simulink model "esquemasi"  (R2020a)
settings: Solver=VariableStepAuto  StartTime=0.0  StopTime=inf  RelTol=1e-3
libraries: simulink x1
settings Model: Creator=TATTO PC  LastModifiedBy=TATTO PC

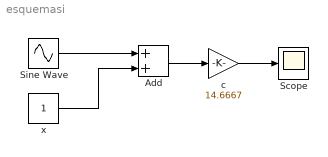
== system esquemasi ==
  Add : Sum
  Scope : Scope
  Sine Wave : Sin  SampleTime=0
  c : Gain  Gain=14.6667
  x : simulink/Math Operations/Slider Gain  gain=1  low=0  high=2
  wires:
  Sine Wave/1 -> Add/1
  Add/1 -> c/1
  c/1 -> Scope/1
  x/1 -> Add/2
